simulink model "Ex5"  (R2020a)
settings: Solver=VariableStepAuto  StartTime=0.0  StopTime=.06  RelTol=1e-3
InitFcn:
  | angle=120; %conduction angle
libraries: powerlib x26
settings Model: Creator=User  LastModifiedBy=User

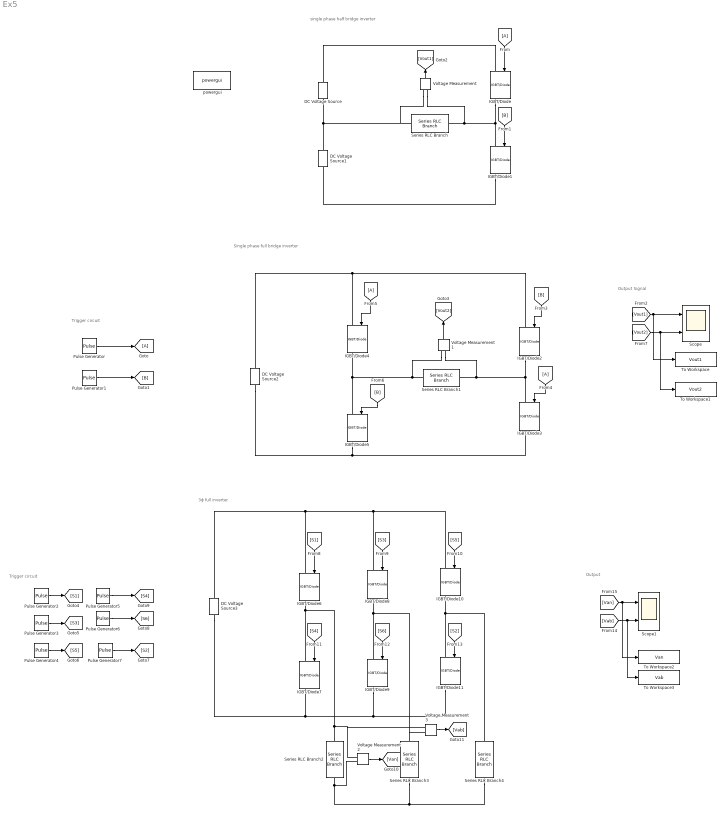
== system Ex5 ==
  note: Output
  note: Trigger circuit
  note: 3ϕ full inverter
  note: Single phase full bridge inverter
  note: Output Signal
  note: Trigger circuit
  note: single phase half bridge inverter
  DC Voltage Source : powerlib/Electrical Sources/DC Voltage Source  Amplitude=50  Measurements=None
  DC Voltage Source1 : powerlib/Electrical Sources/DC Voltage Source  Amplitude=50  Measurements=None
  DC Voltage Source2 : powerlib/Electrical Sources/DC Voltage Source  Amplitude=100  Measurements=None
  DC Voltage Source3 : powerlib/Electrical Sources/DC Voltage Source  Amplitude=100  Measurements=None
  IGBT/Diode{,1..11} (12 alike) : powerlib/Power Electronics/IGBT//Diode  Ron=1e-3  Rs=1e5  Cs=inf  Measurements=on
  Pulse Generator : DiscretePulseGenerator  PulseType=Time based  Period=.02  PulseWidth=50
  Pulse Generator1 : DiscretePulseGenerator  PulseType=Time based  Period=.02  PulseWidth=50  PhaseDelay=.01
  Pulse Generator2 : DiscretePulseGenerator  PulseType=Time based  Period=.02  PulseWidth=(angle/360)*100
  Pulse Generator3 : DiscretePulseGenerator  PulseType=Time based  Period=.02  PulseWidth=(angle/360)*100  PhaseDelay=(120/360)*.02
  Pulse Generator4 : DiscretePulseGenerator  PulseType=Time based  Period=.02  PulseWidth=(angle/360)*100  PhaseDelay=(240/360)*.02
  Pulse Generator5 : DiscretePulseGenerator  PulseType=Time based  Period=.02  PulseWidth=(angle/360)*100  PhaseDelay=(180/360)*.02
  Pulse Generator6 : DiscretePulseGenerator  PulseType=Time based  Period=.02  PulseWidth=(angle/360)*100  PhaseDelay=(300/360)*.02
  Pulse Generator7 : DiscretePulseGenerator  PulseType=Time based  Period=.02  PulseWidth=(angle/360)*100  PhaseDelay=(60/360)*.02
  Scope : Scope  NumInputPorts=2
  Scope1 : Scope  NumInputPorts=2
  Series RLC Branch{,1..4} (5 alike) : powerlib/Elements/Series RLC Branch  LConnTagsString=__new0  RConnTagsString=__new0  BranchType=R  Resistance=1  Inductance=1e-3  SetiL0=off  InitialCurrent=0  Capacitance=1e-6  Setx0=off  InitialVoltage=0  Measurements=None
  To Workspace : ToWorkspace  VariableName=Vout1  SaveFormat=Timeseries  SampleTime=-1
  To Workspace1 : ToWorkspace  VariableName=Vout2  SaveFormat=Timeseries  SampleTime=-1
  To Workspace2 : ToWorkspace  VariableName=Van  SaveFormat=Timeseries  SampleTime=-1
  To Workspace3 : ToWorkspace  VariableName=Vab  SaveFormat=Timeseries  SampleTime=-1
  Voltage Measurement{,1..3} (4 alike) : powerlib/Measurements/Voltage Measurement  PhasorSimulation=off  OutputType=Complex  PSBequivalent=0
  powergui : powerlib/powergui  Priority=1  SimulationMode=Continuous  SampleTime=50e-6  frequency=60  Iterations=50  frequencyindice=0  Pbase=100e6  ErrMax=1e-4  UnitsV=kV  UnitsW=MW  buscounter=0  FunctionMessages=off  echomessages=off  EnableUseOfTLC=off  CurrentSourceSwitches=off  DisableSnubberDevices=on  DisableRonSwitches=on  DisableVfSwitches=on  DisplayEquations=off  AutomaticDiscreteSolvers=off  SolverType=Tustin/Backward Euler (TBE)  Interpol=off  ExternalGateDelay=off  methode=off  Ts=100  x0status=blocks  SPID=on  SwTol=0  HookPort=off  NonlinearTolerance=1e-4  nMaxIteration=100  ContinueOnMaxIteration=off  RestoreLinks=warning  ResistiveCurrentMeasurement=off  Frange=[0:2:500]  Ylog=off  Xlog=on  ShowGrid=off  save=off  variable=ZData  structure=0  ZoomFFT=off  StartTime=0.0  cycles=1  DisplayStyle=1  fundamental=60  FreqAxis=off  MaxFrequency=1000  frequencyindicesteady=1  RmsSteady=1  display=off
  wires:
  Pulse Generator/1 -> [A]
  Pulse Generator1/1 -> [B]
  [A] -> IGBT/Diode/1
  [B] -> IGBT/Diode1/1
  Voltage Measurement/1 -> [Vout1]
  [Vout1] -> To Workspace/1, Scope/1
  [A] -> IGBT/Diode3/1
  [B] -> IGBT/Diode2/1
  Voltage Measurement1/1 -> [Vout2]
  [B] -> IGBT/Diode5/1
  [A] -> IGBT/Diode4/1
  [Vout2] -> To Workspace1/1, Scope/2
  Pulse Generator2/1 -> [S1]
  Pulse Generator3/1 -> [S3]
  Pulse Generator4/1 -> [S5]
  Pulse Generator7/1 -> [S2]
  Pulse Generator6/1 -> [S6]
  Pulse Generator5/1 -> [S4]
  [S1] -> IGBT/Diode6/1
  [S3] -> IGBT/Diode8/1
  [S5] -> IGBT/Diode10/1
  [S4] -> IGBT/Diode7/1
  [S6] -> IGBT/Diode9/1
  [S2] -> IGBT/Diode11/1
  Voltage Measurement2/1 -> [Van]
  Voltage Measurement3/1 -> [Vab]
  [Vab] -> To Workspace3/1, Scope1/2
  [Van] -> To Workspace2/1, Scope1/1
  connections:
  DC Voltage Source1/RConn1 -- Voltage Measurement/LConn1 -- Series RLC Branch/LConn1 -- DC Voltage Source/LConn1
  IGBT/Diode/RConn1 -- IGBT/Diode1/LConn1 -- Voltage Measurement/LConn2 -- Series RLC Branch/RConn1
  IGBT/Diode1/RConn1 -- DC Voltage Source1/LConn1
  DC Voltage Source/RConn1 -- IGBT/Diode/LConn1
  IGBT/Diode4/LConn1 -- DC Voltage Source2/RConn1 -- IGBT/Diode2/LConn1
  IGBT/Diode5/RConn1 -- DC Voltage Source2/LConn1 -- IGBT/Diode3/RConn1
  IGBT/Diode3/LConn1 -- IGBT/Diode2/RConn1 -- Voltage Measurement1/LConn2 -- Series RLC Branch1/RConn1
  Series RLC Branch1/LConn1 -- Voltage Measurement1/LConn1 -- IGBT/Diode4/RConn1 -- IGBT/Diode5/LConn1
  IGBT/Diode7/LConn1 -- Voltage Measurement2/LConn1 -- Voltage Measurement3/LConn1 -- Series RLC Branch2/LConn1 -- IGBT/Diode6/RConn1
  IGBT/Diode9/LConn1 -- Voltage Measurement3/LConn2 -- Series RLC Branch3/LConn1 -- IGBT/Diode8/RConn1
  IGBT/Diode11/LConn1 -- Series RLC Branch4/LConn1 -- IGBT/Diode10/RConn1
  IGBT/Diode10/LConn1 -- IGBT/Diode8/LConn1 -- DC Voltage Source3/RConn1 -- IGBT/Diode6/LConn1
  IGBT/Diode11/RConn1 -- IGBT/Diode9/RConn1 -- DC Voltage Source3/LConn1 -- IGBT/Diode7/RConn1
  Series RLC Branch4/RConn1 -- Series RLC Branch3/RConn1 -- Voltage Measurement2/LConn2 -- Series RLC Branch2/RConn1
